simulink model "ASM_Traffic_V2X_Complete_Model_2"  (R2019a)
settings: Solver=ode1  StartTime=SIM.tstart.v  StopTime=Inf  FixedStep=SIM.StepSize.v  RelTol=1e-3
PostLoadFcn:
  | if any(exist('dsrtsu_mdlpostloadfcn', 'file') ~= 0), dsrtsu_mdlpostloadfcn('Execute', bdroot); end
  | try, asm_mdl_postloadfcn(bdroot, 'UpdateModel', 2200); catch, disp(lasterr); end,
undefined symbols (not defined in the file): _SensorPnts_1, _SensorPnts_13, _SensorPnts_17, _SensorPnts_21, _SensorPnts_25, _SensorPnts_29, _SensorPnts_33, _SensorPnts_37, _SensorPnts_41, _SensorPnts_45, _SensorPnts_49, _SensorPnts_5, _SensorPnts_53, _SensorPnts_57, _SensorPnts_9, _to_, CPT, G5A, ITS, MDL, rad, s_to_rpm, SIM
libraries: simulink x169, ASM_VehicleDynamics_lib x126, ASM_Traffic_lib x83, ASM_Utils_lib x49, mdbs x45, ASM_Environment_lib x17, dspindex x12, dsaV2xLibraryAux x10, dsmpblib x6, dsaV2xAsn1Library x4, dsaV2xLibrary x4, ASM_BrakeHydraulics_lib x4
(part 29 of 36)

== system ASM_Traffic_V2X_Complete_Model_2/MDL/Environment/Traffic/Sensors/Object_Sensor_3D/SensorMapping/NearestSurfaceMapping ==
  Sensor1_Signals[] : Inport
  Sensor2_Signals[] : Inport  Port=2
  Sensor3_Signals[] : Inport  Port=3
  NearestSurfaceSignals_Sensor1 : Subsystem
  NearestSurfaceSignals_Sensor2 : Subsystem
  NearestSurfaceSignals_Sensor3 : Subsystem
  Terminator{1..42} (42 alike) : Terminator
  wires:
  NearestSurfaceSignals_Sensor1/10(Pos_x_NearstSurfacePnt4_CoorSys_S[m]) -> Terminator42/1
  NearestSurfaceSignals_Sensor1/8(Pos_y_NearstSurfacePnt3_CoorSys_S[m]) -> Terminator12/1
  NearestSurfaceSignals_Sensor1/7(Pos_x_NearstSurfacePnt3_CoorSys_S[m]) -> Terminator11/1
  NearestSurfaceSignals_Sensor1/12(Pos_z_NearstSurfacePnt4_CoorSys_S[m]) -> Terminator4/1
  NearestSurfaceSignals_Sensor1/9(Pos_z_NearstSurfacePnt3_CoorSys_S[m]) -> Terminator13/1
  NearestSurfaceSignals_Sensor1/11(Pos_y_NearstSurfacePnt4_CoorSys_S[m]) -> Terminator3/1
  NearestSurfaceSignals_Sensor1/13(NearestSurf_Pnts_Index[]) -> Terminator5/1
  NearestSurfaceSignals_Sensor1/14(NearestSurf_Index[]) -> Terminator6/1
  NearestSurfaceSignals_Sensor1/1(Pos_x_NearstSurfacePnt1_CoorSys_S[m]) -> Terminator1/1
  NearestSurfaceSignals_Sensor1/6(Pos_z_NearstSurfacePnt2_CoorSys_S[m]) -> Terminator10/1
  NearestSurfaceSignals_Sensor1/5(Pos_y_NearstSurfacePnt2_CoorSys_S[m]) -> Terminator9/1
  NearestSurfaceSignals_Sensor1/2(Pos_y_NearstSurfacePnt1_CoorSys_S[m]) -> Terminator2/1
  NearestSurfaceSignals_Sensor1/4(Pos_x_NearstSurfacePnt2_CoorSys_S[m]) -> Terminator8/1
  NearestSurfaceSignals_Sensor1/3(Pos_z_NearstSurfacePnt1_CoorSys_S[m]) -> Terminator7/1
  NearestSurfaceSignals_Sensor3/10(Pos_x_NearstSurfacePnt4_CoorSys_S[m]) -> Terminator41/1
  NearestSurfaceSignals_Sensor3/8(Pos_y_NearstSurfacePnt3_CoorSys_S[m]) -> Terminator39/1
  NearestSurfaceSignals_Sensor3/7(Pos_x_NearstSurfacePnt3_CoorSys_S[m]) -> Terminator38/1
  NearestSurfaceSignals_Sensor3/12(Pos_z_NearstSurfacePnt4_CoorSys_S[m]) -> Terminator31/1
  NearestSurfaceSignals_Sensor3/9(Pos_z_NearstSurfacePnt3_CoorSys_S[m]) -> Terminator40/1
  NearestSurfaceSignals_Sensor3/11(Pos_y_NearstSurfacePnt4_CoorSys_S[m]) -> Terminator30/1
  NearestSurfaceSignals_Sensor3/13(NearestSurf_Pnts_Index[]) -> Terminator32/1
  NearestSurfaceSignals_Sensor3/14(NearestSurf_Index[]) -> Terminator33/1
  NearestSurfaceSignals_Sensor3/1(Pos_x_NearstSurfacePnt1_CoorSys_S[m]) -> Terminator28/1
  NearestSurfaceSignals_Sensor3/6(Pos_z_NearstSurfacePnt2_CoorSys_S[m]) -> Terminator37/1
  NearestSurfaceSignals_Sensor3/5(Pos_y_NearstSurfacePnt2_CoorSys_S[m]) -> Terminator36/1
  NearestSurfaceSignals_Sensor3/2(Pos_y_NearstSurfacePnt1_CoorSys_S[m]) -> Terminator29/1
  NearestSurfaceSignals_Sensor3/4(Pos_x_NearstSurfacePnt2_CoorSys_S[m]) -> Terminator35/1
  NearestSurfaceSignals_Sensor3/3(Pos_z_NearstSurfacePnt1_CoorSys_S[m]) -> Terminator34/1
  NearestSurfaceSignals_Sensor2/3(Pos_z_NearstSurfacePnt1_CoorSys_S[m]) -> Terminator20/1
  NearestSurfaceSignals_Sensor2/4(Pos_x_NearstSurfacePnt2_CoorSys_S[m]) -> Terminator21/1
  NearestSurfaceSignals_Sensor2/2(Pos_y_NearstSurfacePnt1_CoorSys_S[m]) -> Terminator15/1
  NearestSurfaceSignals_Sensor2/5(Pos_y_NearstSurfacePnt2_CoorSys_S[m]) -> Terminator22/1
  NearestSurfaceSignals_Sensor2/6(Pos_z_NearstSurfacePnt2_CoorSys_S[m]) -> Terminator23/1
  NearestSurfaceSignals_Sensor2/1(Pos_x_NearstSurfacePnt1_CoorSys_S[m]) -> Terminator14/1
  NearestSurfaceSignals_Sensor2/14(NearestSurf_Index[]) -> Terminator19/1
  NearestSurfaceSignals_Sensor2/13(NearestSurf_Pnts_Index[]) -> Terminator18/1
  Sensor2_Signals[]/1 -> NearestSurfaceSignals_Sensor2/1(SensorSignals[])
  Sensor3_Signals[]/1 -> NearestSurfaceSignals_Sensor3/1(SensorSignals[])
  Sensor1_Signals[]/1 -> NearestSurfaceSignals_Sensor1/1(SensorSignals[])
  NearestSurfaceSignals_Sensor2/11(Pos_y_NearstSurfacePnt4_CoorSys_S[m]) -> Terminator16/1
  NearestSurfaceSignals_Sensor2/9(Pos_z_NearstSurfacePnt3_CoorSys_S[m]) -> Terminator26/1
  NearestSurfaceSignals_Sensor2/12(Pos_z_NearstSurfacePnt4_CoorSys_S[m]) -> Terminator17/1
  NearestSurfaceSignals_Sensor2/7(Pos_x_NearstSurfacePnt3_CoorSys_S[m]) -> Terminator24/1
  NearestSurfaceSignals_Sensor2/8(Pos_y_NearstSurfacePnt3_CoorSys_S[m]) -> Terminator25/1
  NearestSurfaceSignals_Sensor2/10(Pos_x_NearstSurfacePnt4_CoorSys_S[m]) -> Terminator27/1

== system ASM_Traffic_V2X_Complete_Model_2/MDL/Environment/Traffic/Sensors/Object_Sensor_3D/SensorMapping/Signals_to_ACC_SoftECU ==
  Sensor_1_ACC_In : Inport
  Sensor_2_ACC_In : Inport  Port=2
  Bus Creator : BusCreator  Inputs=3
  Bus Creator1 : BusCreator  Inputs=2
  Bus Creator2 : BusCreator  Inputs=4
  Bus Selector : BusSelector  OutputSignals=SensorOutput.Dist_Object[m],SensorOutput.v_Rel_Object[m|s],SensorOutput.Angle_Hor_Object[deg]
  Bus Selector1 : BusSelector  OutputSignals=SensorOutput.Dist_Object[m],SensorOutput.v_Rel_Object[m|s],SensorOutput.Angle_Hor_Object[deg],SensorOutput.Object_ID[]
  Sensor_Signals : Outport
  wires:
  Bus Selector1/3 -> Bus Creator2/3  "<Angle_Hor_Object[deg]>"
  Bus Selector1/2 -> Bus Creator2/2  "<v_Rel_Object[m|s]>"
  Sensor_2_ACC_In/1 -> Bus Selector1/1
  Bus Selector1/4 -> Bus Creator2/4  "<Object_ID[]>"
  Bus Selector1/1 -> Bus Creator2/1  "<Dist_Object[m]>"
  Bus Creator2/1 -> Bus Creator1/2  "Sensor_2_ACC"
  Sensor_1_ACC_In/1 -> Bus Selector/1
  Bus Selector/1 -> Bus Creator/1  "<Dist_Object[m]>"
  Bus Selector/2 -> Bus Creator/2  "<v_Rel_Object[m|s]>"
  Bus Selector/3 -> Bus Creator/3  "<Angle_Hor_Object[deg]>"
  Bus Creator/1 -> Bus Creator1/1  "Sensor_1_ACC"
  Bus Creator1/1 -> Sensor_Signals/1  "SensorSignals"

== system ASM_Traffic_V2X_Complete_Model_2/MDL/Environment/Traffic/Sensors/Object_Sensor_3D/SensorParameters/ObjectSensor3DParameters_1 ==
  Demux : Demux  Outputs=3
  Demux1 : Demux  Outputs=3
  MODELDESK_GROUP : ASM_Utils_lib/ModelDeskInterface/MODELDESK_GROUP  MDLDGroup=Object Sensor 3D 1  ASMProperties=struct('Name','MODELDESK_GROUP','Version','1.0','Library','ASM_Utils_lib')
  Mux1 : Mux  Inputs=21
  OBJECT_SENSOR_3D_PARAMETERS_1 : ASM_Traffic_lib/Sensors/Object_Sensor_3D/OBJECT_SENSOR_3D_PARAMETERS  Tag=ASM_SUBCOMPONENT  Sw_Sensor_Enable=MDL.Traffic.Sensors.ObjectSensor3D_1.Sw_Sensor_Enable  Const_SensorIdx=MDL.Traffic.Sensors.ObjectSensor3D_1.Const_SensorIdx  Const_t_Offs_Sensor=MDL.Traffic.Sensors.ObjectSensor3D_1.Const_t_Offs_Sensor  Const_t_Cycle_Sensor=MDL.Traffic.Sensors.ObjectSensor3D_1.Const_t_Cycle_Sensor  Const_t_Delay_SensorOutput=MDL.Traffic.Sensors.ObjectSensor3D_1.Const_t_Delay_SensorOutput  Sw_Geometry=MDL.Traffic.Sensors.ObjectSensor3D_1.Sw_Geometry  Const_Pos_Sensor_Apex_CoorSys_V=MDL.Traffic.Sensors.ObjectSensor3D_1.Const_Pos_Sensor_Apex_CoorSys_V  Const_Angle_Orientation_Sensor_CoorSys_V=MDL.Traffic.Sensors.ObjectSensor3D_1.Const_Angle_Orientation_Sensor_CoorSys_V  Const_Length_ScopeZone=MDL.Traffic.Sensors.ObjectSensor3D_1.Const_Length_ScopeZone  Const_Angle_ScopeZone_Horizontal=MDL.Traffic.Sensors.ObjectSensor3D_1.Const_Angle_ScopeZone_Horizontal  Const_Angle_ScopeZone_Vertical=MDL.Traffic.Sensors.ObjectSensor3D_1.Const_Angle_ScopeZone_Vertical  Const_Length_ScopeZone_Head=MDL.Traffic.Sensors.ObjectSensor3D_1.Const_Length_ScopeZone_Head  Const_Length_BlindZone=MDL.Traffic.Sensors.ObjectSensor3D_1.Const_Length_BlindZone  Sw_Occlusion_Mode=MDL.Traffic.Sensors.ObjectSensor3D_1.Sw_Occlusion_Mode  Const_Threshold_Occlusion_Ratio=MDL.Traffic.Sensors.ObjectSensor3D_1.Const_Threshold_Occlusion_Ratio  Sw_Object_Points_Calculation_Enable=MDL.Traffic.Sensors.ObjectSensor3D_1.Sw_Object_Points_Calculation_Enable  Sw_Object_Points_Occlusion_Enable=MDL.Traffic.Sensors.ObjectSensor3D_1.Sw_Object_Points_Occlusion_Enable  ASMProperties=struct('Name','OBJECT_SENSOR_3D_PARAMETERS','Version','4.0','Library','ASM_Traffic_lib')  ASMInstanceName=object_sensor_3d_parameters  ASMInstanceID=1
  Sensor_Parameters[] : Outport
  tag scope: ASMBUS_Environment_Traffic_3DObjSensor1_Parameters=global
  wires:
  OBJECT_SENSOR_3D_PARAMETERS_1/18 -> Mux1/21
  OBJECT_SENSOR_3D_PARAMETERS_1/17 -> Mux1/20
  OBJECT_SENSOR_3D_PARAMETERS_1/16 -> Mux1/19
  OBJECT_SENSOR_3D_PARAMETERS_1/15 -> Mux1/18
  Demux1/3 -> Mux1/12
  Demux1/1 -> Mux1/10
  Demux1/2 -> Mux1/11
  Demux/3 -> Mux1/9
  Demux/2 -> Mux1/8
  Demux/1 -> Mux1/7
  OBJECT_SENSOR_3D_PARAMETERS_1/14 -> Mux1/17
  OBJECT_SENSOR_3D_PARAMETERS_1/11 -> Mux1/14
  OBJECT_SENSOR_3D_PARAMETERS_1/6 -> Mux1/5
  OBJECT_SENSOR_3D_PARAMETERS_1/5 -> Mux1/4
  OBJECT_SENSOR_3D_PARAMETERS_1/4 -> Mux1/3
  Mux1/1 -> Sensor_Parameters[]/1
  OBJECT_SENSOR_3D_PARAMETERS_1/10 -> Mux1/13
  OBJECT_SENSOR_3D_PARAMETERS_1/13 -> Mux1/16
  OBJECT_SENSOR_3D_PARAMETERS_1/9 -> Demux1/1
  OBJECT_SENSOR_3D_PARAMETERS_1/8 -> Demux/1
  OBJECT_SENSOR_3D_PARAMETERS_1/1 -> [ASMBUS_Environment_Traffic_3DObjSensor1_Parameters]
  OBJECT_SENSOR_3D_PARAMETERS_1/3 -> Mux1/2
  OBJECT_SENSOR_3D_PARAMETERS_1/2 -> Mux1/1
  OBJECT_SENSOR_3D_PARAMETERS_1/12 -> Mux1/15
  OBJECT_SENSOR_3D_PARAMETERS_1/7 -> Mux1/6

== system ASM_Traffic_V2X_Complete_Model_2/MDL/Environment/Traffic/Sensors/Object_Sensor_3D/SensorParameters/ObjectSensor3DParameters_2 ==
  Demux2 : Demux  Outputs=3
  Demux3 : Demux  Outputs=3
  MODELDESK_GROUP : ASM_Utils_lib/ModelDeskInterface/MODELDESK_GROUP  MDLDGroup=Object Sensor 3D 2  ASMProperties=struct('Name','MODELDESK_GROUP','Version','1.0','Library','ASM_Utils_lib')
  Mux : Mux  Inputs=21
  OBJECT_SENSOR_3D_PARAMETERS_2 : ASM_Traffic_lib/Sensors/Object_Sensor_3D/OBJECT_SENSOR_3D_PARAMETERS  Tag=ASM_SUBCOMPONENT  Sw_Sensor_Enable=MDL.Traffic.Sensors.ObjectSensor3D_2.Sw_Sensor_Enable  Const_SensorIdx=MDL.Traffic.Sensors.ObjectSensor3D_2.Const_SensorIdx  Const_t_Offs_Sensor=MDL.Traffic.Sensors.ObjectSensor3D_2.Const_t_Offs_Sensor  Const_t_Cycle_Sensor=MDL.Traffic.Sensors.ObjectSensor3D_2.Const_t_Cycle_Sensor  Const_t_Delay_SensorOutput=MDL.Traffic.Sensors.ObjectSensor3D_2.Const_t_Delay_SensorOutput  Sw_Geometry=MDL.Traffic.Sensors.ObjectSensor3D_2.Sw_Geometry  Const_Pos_Sensor_Apex_CoorSys_V=MDL.Traffic.Sensors.ObjectSensor3D_2.Const_Pos_Sensor_Apex_CoorSys_V  Const_Angle_Orientation_Sensor_CoorSys_V=MDL.Traffic.Sensors.ObjectSensor3D_2.Const_Angle_Orientation_Sensor_CoorSys_V  Const_Length_ScopeZone=MDL.Traffic.Sensors.ObjectSensor3D_2.Const_Length_ScopeZone  Const_Angle_ScopeZone_Horizontal=MDL.Traffic.Sensors.ObjectSensor3D_2.Const_Angle_ScopeZone_Horizontal  Const_Angle_ScopeZone_Vertical=MDL.Traffic.Sensors.ObjectSensor3D_2.Const_Angle_ScopeZone_Vertical  Const_Length_ScopeZone_Head=MDL.Traffic.Sensors.ObjectSensor3D_2.Const_Length_ScopeZone_Head  Const_Length_BlindZone=MDL.Traffic.Sensors.ObjectSensor3D_2.Const_Length_BlindZone  Sw_Occlusion_Mode=MDL.Traffic.Sensors.ObjectSensor3D_2.Sw_Occlusion_Mode  Const_Threshold_Occlusion_Ratio=MDL.Traffic.Sensors.ObjectSensor3D_2.Const_Threshold_Occlusion_Ratio  Sw_Object_Points_Calculation_Enable=MDL.Traffic.Sensors.ObjectSensor3D_2.Sw_Object_Points_Calculation_Enable  Sw_Object_Points_Occlusion_Enable=MDL.Traffic.Sensors.ObjectSensor3D_2.Sw_Object_Points_Occlusion_Enable  ASMProperties=struct('Name','OBJECT_SENSOR_3D_PARAMETERS','Version','4.0','Library','ASM_Traffic_lib')  ASMInstanceName=object_sensor_3d_parameters  ASMInstanceID=2
      settings: AttributesFormatString=Instance Name: object_sensor_3d_parameters\nInstance ID: 2
  Sensor_Parameters[] : Outport
  tag scope: ASMBUS_Environment_Traffic_3DObjSensor2_Parameters=global
  wires:
  OBJECT_SENSOR_3D_PARAMETERS_2/18 -> Mux/21
  OBJECT_SENSOR_3D_PARAMETERS_2/17 -> Mux/20
  OBJECT_SENSOR_3D_PARAMETERS_2/16 -> Mux/19
  OBJECT_SENSOR_3D_PARAMETERS_2/15 -> Mux/18
  Demux3/3 -> Mux/12
  Demux3/1 -> Mux/10
  Demux3/2 -> Mux/11
  Demux2/3 -> Mux/9
  Demux2/1 -> Mux/7
  Demux2/2 -> Mux/8
  Mux/1 -> Sensor_Parameters[]/1
  OBJECT_SENSOR_3D_PARAMETERS_2/14 -> Mux/17
  OBJECT_SENSOR_3D_PARAMETERS_2/12 -> Mux/15
  OBJECT_SENSOR_3D_PARAMETERS_2/1 -> [ASMBUS_Environment_Traffic_3DObjSensor2_Parameters]
  OBJECT_SENSOR_3D_PARAMETERS_2/9 -> Demux3/1
  OBJECT_SENSOR_3D_PARAMETERS_2/10 -> Mux/13
  OBJECT_SENSOR_3D_PARAMETERS_2/3 -> Mux/2
  OBJECT_SENSOR_3D_PARAMETERS_2/7 -> Mux/6
  OBJECT_SENSOR_3D_PARAMETERS_2/4 -> Mux/3
  OBJECT_SENSOR_3D_PARAMETERS_2/13 -> Mux/16
  OBJECT_SENSOR_3D_PARAMETERS_2/8 -> Demux2/1
  OBJECT_SENSOR_3D_PARAMETERS_2/6 -> Mux/5
  OBJECT_SENSOR_3D_PARAMETERS_2/11 -> Mux/14
  OBJECT_SENSOR_3D_PARAMETERS_2/2 -> Mux/1
  OBJECT_SENSOR_3D_PARAMETERS_2/5 -> Mux/4

== system ASM_Traffic_V2X_Complete_Model_2/MDL/Environment/Traffic/Sensors/Object_Sensor_3D/SensorParameters/ObjectSensor3DParameters_3 ==
  Demux4 : Demux  Outputs=3
  Demux5 : Demux  Outputs=3
  MODELDESK_GROUP : ASM_Utils_lib/ModelDeskInterface/MODELDESK_GROUP  MDLDGroup=Object Sensor 3D 3  ASMProperties=struct('Name','MODELDESK_GROUP','Version','1.0','Library','ASM_Utils_lib')
  Mux2 : Mux  Inputs=21
  OBJECT_SENSOR_3D_PARAMETERS_3 : ASM_Traffic_lib/Sensors/Object_Sensor_3D/OBJECT_SENSOR_3D_PARAMETERS  Tag=ASM_SUBCOMPONENT  Sw_Sensor_Enable=MDL.Traffic.Sensors.ObjectSensor3D_3.Sw_Sensor_Enable  Const_SensorIdx=MDL.Traffic.Sensors.ObjectSensor3D_3.Const_SensorIdx  Const_t_Offs_Sensor=MDL.Traffic.Sensors.ObjectSensor3D_3.Const_t_Offs_Sensor  Const_t_Cycle_Sensor=MDL.Traffic.Sensors.ObjectSensor3D_3.Const_t_Cycle_Sensor  Const_t_Delay_SensorOutput=MDL.Traffic.Sensors.ObjectSensor3D_3.Const_t_Delay_SensorOutput  Sw_Geometry=MDL.Traffic.Sensors.ObjectSensor3D_3.Sw_Geometry  Const_Pos_Sensor_Apex_CoorSys_V=MDL.Traffic.Sensors.ObjectSensor3D_3.Const_Pos_Sensor_Apex_CoorSys_V  Const_Angle_Orientation_Sensor_CoorSys_V=MDL.Traffic.Sensors.ObjectSensor3D_3.Const_Angle_Orientation_Sensor_CoorSys_V  Const_Length_ScopeZone=MDL.Traffic.Sensors.ObjectSensor3D_3.Const_Length_ScopeZone  Const_Angle_ScopeZone_Horizontal=MDL.Traffic.Sensors.ObjectSensor3D_3.Const_Angle_ScopeZone_Horizontal  Const_Angle_ScopeZone_Vertical=MDL.Traffic.Sensors.ObjectSensor3D_3.Const_Angle_ScopeZone_Vertical  Const_Length_ScopeZone_Head=MDL.Traffic.Sensors.ObjectSensor3D_3.Const_Length_ScopeZone_Head  Const_Length_BlindZone=MDL.Traffic.Sensors.ObjectSensor3D_3.Const_Length_BlindZone  Sw_Occlusion_Mode=MDL.Traffic.Sensors.ObjectSensor3D_3.Sw_Occlusion_Mode  Const_Threshold_Occlusion_Ratio=MDL.Traffic.Sensors.ObjectSensor3D_3.Const_Threshold_Occlusion_Ratio  Sw_Object_Points_Calculation_Enable=MDL.Traffic.Sensors.ObjectSensor3D_3.Sw_Object_Points_Calculation_Enable  Sw_Object_Points_Occlusion_Enable=MDL.Traffic.Sensors.ObjectSensor3D_3.Sw_Object_Points_Occlusion_Enable  ASMProperties=struct('Name','OBJECT_SENSOR_3D_PARAMETERS','Version','4.0','Library','ASM_Traffic_lib')  ASMInstanceName=object_sensor_3d_parameters  ASMInstanceID=3
      settings: AttributesFormatString=Instance Name: object_sensor_3d_parameters\nInstance ID: 3
  Sensor_Parameters[] : Outport
  tag scope: ASMBUS_Environment_Traffic_3DObjSensor3_Parameters=global
  wires:
  OBJECT_SENSOR_3D_PARAMETERS_3/18 -> Mux2/21
  OBJECT_SENSOR_3D_PARAMETERS_3/17 -> Mux2/20
  OBJECT_SENSOR_3D_PARAMETERS_3/16 -> Mux2/19
  OBJECT_SENSOR_3D_PARAMETERS_3/15 -> Mux2/18
  Demux5/3 -> Mux2/9
  Demux5/1 -> Mux2/7
  Demux5/2 -> Mux2/8
  Demux4/3 -> Mux2/12
  Demux4/1 -> Mux2/10
  Demux4/2 -> Mux2/11
  Mux2/1 -> Sensor_Parameters[]/1
  OBJECT_SENSOR_3D_PARAMETERS_3/14 -> Mux2/17
  OBJECT_SENSOR_3D_PARAMETERS_3/13 -> Mux2/16
  OBJECT_SENSOR_3D_PARAMETERS_3/12 -> Mux2/15
  OBJECT_SENSOR_3D_PARAMETERS_3/11 -> Mux2/14
  OBJECT_SENSOR_3D_PARAMETERS_3/10 -> Mux2/13
  OBJECT_SENSOR_3D_PARAMETERS_3/9 -> Demux4/1
  OBJECT_SENSOR_3D_PARAMETERS_3/8 -> Demux5/1
  OBJECT_SENSOR_3D_PARAMETERS_3/7 -> Mux2/6
  OBJECT_SENSOR_3D_PARAMETERS_3/6 -> Mux2/5
  OBJECT_SENSOR_3D_PARAMETERS_3/5 -> Mux2/4
  OBJECT_SENSOR_3D_PARAMETERS_3/4 -> Mux2/3
  OBJECT_SENSOR_3D_PARAMETERS_3/3 -> Mux2/2
  OBJECT_SENSOR_3D_PARAMETERS_3/2 -> Mux2/1
  OBJECT_SENSOR_3D_PARAMETERS_3/1 -> [ASMBUS_Environment_Traffic_3DObjSensor3_Parameters]

== system ASM_Traffic_V2X_Complete_Model_2/MDLUserInterface/Environment/MDL_DISP/Traffic/Fellow_Movement/GetFellowDataByIndex_1/SwitchFellowMovementData ==
  TrafficBus : Inport
  Switch : Inport  Port=2
  Bus Selector2 : BusSelector  OutputSignals=FellowMovement.TrafficScheduler.Flag_FellowsUsed[0|1]
  Bus Selector3 : BusSelector  OutputSignals=FellowMovement.FellowMovement.s_Fellows[m]
  Bus Selector4 : BusSelector  OutputSignals=FellowMovement.FellowMovement.d_Total_Fellows[m]
  Bus Selector5 : BusSelector  OutputSignals=FellowMovement.FellowMovement.v_Fellows[km|h]
  Flag_Fellow_Used[0|1] : Subsystem
      mask Display: disp('')
  Selector{,1..3} (4 alike) : Selector  InputPortWidth=MDL.Traffic.MaxNumFellows.v  IndexOptions=Index vector (port)  Indices=[1 3]  OutputSizes=1
  d_Total_Fellow[m] : Subsystem
      mask Display: disp('')
  s_Fellow[m] : Subsystem
      mask Display: disp('')
  v_Fellow[km|h] : Subsystem
      mask Display: disp('')
  "Flag_Fellow_Used[0|1] " : Outport
  "s_Fellow[m] " : Outport  Port=2
  "d_Total_Fellow[m] " : Outport  Port=3
  "v_Fellow[km|h] " : Outport  Port=4
  wires:
  Flag_Fellow_Used[0|1]/1(Out1) -> "Flag_Fellow_Used[0|1] "/1  "Flag_Fellow_Used[0|1]"
  s_Fellow[m]/1(Out1) -> "s_Fellow[m] "/1  "s_Fellow[m]"
  d_Total_Fellow[m]/1(Out1) -> "d_Total_Fellow[m] "/1  "d_Total_Fellow[m]"
  v_Fellow[km|h]/1(Out1) -> "v_Fellow[km|h] "/1  "v_Fellow[km|h]"
  Switch/1 -> Selector3/2, Selector2/2, Selector1/2, Selector/2
  Bus Selector2/1 -> Selector/1  "<Flag_FellowsUsed[0|1]>"
  Selector/1 -> Flag_Fellow_Used[0|1]/1(In1)
  Bus Selector3/1 -> Selector1/1  "<s_Fellows[m]>"
  Selector1/1 -> s_Fellow[m]/1(In1)
  Bus Selector4/1 -> Selector2/1  "<d_Total_Fellows[m]>"
  Selector2/1 -> d_Total_Fellow[m]/1(In1)
  Bus Selector5/1 -> Selector3/1  "<v_Fellows[km|h]>"
  Selector3/1 -> v_Fellow[km|h]/1(In1)
  TrafficBus/1 -> Bus Selector5/1, Bus Selector4/1, Bus Selector3/1, Bus Selector2/1

== system ASM_Traffic_V2X_Complete_Model_2/MDLUserInterface/Environment/MDL_DISP/Traffic/Fellow_Movement/GetFellowDataByIndex_1/SwitchInfoData ==
  TrafficBus : Inport
  Switch : Inport  Port=2
  Bus Selector1 : BusSelector  OutputSignals=FellowMovement.TrafficScheduler.Info.CurrentSegment_Fellows[]
  Bus Selector2 : BusSelector  OutputSignals=FellowMovement.TrafficScheduler.Info.t_local_Fellows[s]
  Bus Selector44 : BusSelector  OutputSignals=FellowMovement.TrafficScheduler.Info.CurrentSequence_Fellows[]
  Selector : Selector  InputPortWidth=MDL.Traffic.MaxNumFellows.v  IndexOptions=Index vector (port)  Indices=[1 3]  OutputSizes=1
  Selector1 : Selector  InputPortWidth=MDL.Traffic.MaxNumFellows.v  IndexOptions=Index vector (port)  Indices=[1 3]  OutputSizes=1
  Selector2 : Selector  InputPortWidth=MDL.Traffic.MaxNumFellows.v  IndexOptions=Index vector (port)  Indices=[1 3]  OutputSizes=1
  CurrentSequence[] : Outport
  CurrentSegment[] : Outport  Port=2
  t_local[s] : Outport  Port=3
  wires:
  Bus Selector2/1 -> Selector2/1  "<t_local_Fellows[s]>"
  TrafficBus/1 -> Bus Selector2/1, Bus Selector1/1, Bus Selector44/1
  Bus Selector1/1 -> Selector1/1  "<CurrentSegment_Fellows[]>"
  Selector1/1 -> CurrentSegment[]/1
  Bus Selector44/1 -> Selector/1  "<CurrentSequence_Fellows[]>"
  Selector/1 -> CurrentSequence[]/1
  Switch/1 -> Selector2/2, Selector1/2, Selector/2
  Selector2/1 -> t_local[s]/1

== system ASM_Traffic_V2X_Complete_Model_2/MDLUserInterface/Environment/MDL_DISP/Traffic/Fellow_Movement/GetFellowDataByIndex_2/SwitchFellowMovementData ==
  TrafficBus : Inport
  Switch : Inport  Port=2
  Bus Selector2 : BusSelector  OutputSignals=FellowMovement.TrafficScheduler.Flag_FellowsUsed[0|1]
  Bus Selector3 : BusSelector  OutputSignals=FellowMovement.FellowMovement.s_Fellows[m]
  Bus Selector4 : BusSelector  OutputSignals=FellowMovement.FellowMovement.d_Total_Fellows[m]
  Bus Selector5 : BusSelector  OutputSignals=FellowMovement.FellowMovement.v_Fellows[km|h]
  Flag_Fellow_Used[0|1] : Subsystem
      mask Display: disp('')
  Selector{,1..3} (4 alike) : Selector  InputPortWidth=MDL.Traffic.MaxNumFellows.v  IndexOptions=Index vector (port)  Indices=[1 3]  OutputSizes=1
  d_Total_Fellow[m] : Subsystem
      mask Display: disp('')
  s_Fellow[m] : Subsystem
      mask Display: disp('')
  v_Fellow[km|h] : Subsystem
      mask Display: disp('')
  "Flag_Fellow_Used[0|1] " : Outport
  "s_Fellow[m] " : Outport  Port=2
  "d_Total_Fellow[m] " : Outport  Port=3
  "v_Fellow[km|h] " : Outport  Port=4
  wires:
  TrafficBus/1 -> Bus Selector2/1, Bus Selector3/1, Bus Selector4/1, Bus Selector5/1
  Selector3/1 -> v_Fellow[km|h]/1(In1)
  Bus Selector5/1 -> Selector3/1  "<v_Fellows[km|h]>"
  Selector2/1 -> d_Total_Fellow[m]/1(In1)
  Bus Selector4/1 -> Selector2/1  "<d_Total_Fellows[m]>"
  Selector1/1 -> s_Fellow[m]/1(In1)
  Bus Selector3/1 -> Selector1/1  "<s_Fellows[m]>"
  Selector/1 -> Flag_Fellow_Used[0|1]/1(In1)
  Bus Selector2/1 -> Selector/1  "<Flag_FellowsUsed[0|1]>"
  Switch/1 -> Selector/2, Selector1/2, Selector2/2, Selector3/2
  v_Fellow[km|h]/1(Out1) -> "v_Fellow[km|h] "/1  "v_Fellow[km|h]"
  d_Total_Fellow[m]/1(Out1) -> "d_Total_Fellow[m] "/1  "d_Total_Fellow[m]"
  s_Fellow[m]/1(Out1) -> "s_Fellow[m] "/1  "s_Fellow[m]"
  Flag_Fellow_Used[0|1]/1(Out1) -> "Flag_Fellow_Used[0|1] "/1  "Flag_Fellow_Used[0|1]"

== system ASM_Traffic_V2X_Complete_Model_2/MDLUserInterface/Environment/MDL_DISP/Traffic/Fellow_Movement/GetFellowDataByIndex_2/SwitchInfoData ==
  TrafficBus : Inport
  Switch : Inport  Port=2
  Bus Selector1 : BusSelector  OutputSignals=FellowMovement.TrafficScheduler.Info.CurrentSegment_Fellows[]
  Bus Selector2 : BusSelector  OutputSignals=FellowMovement.TrafficScheduler.Info.t_local_Fellows[s]
  Bus Selector44 : BusSelector  OutputSignals=FellowMovement.TrafficScheduler.Info.CurrentSequence_Fellows[]
  Selector : Selector  InputPortWidth=MDL.Traffic.MaxNumFellows.v  IndexOptions=Index vector (port)  Indices=[1 3]  OutputSizes=1
  Selector1 : Selector  InputPortWidth=MDL.Traffic.MaxNumFellows.v  IndexOptions=Index vector (port)  Indices=[1 3]  OutputSizes=1
  Selector2 : Selector  InputPortWidth=MDL.Traffic.MaxNumFellows.v  IndexOptions=Index vector (port)  Indices=[1 3]  OutputSizes=1
  CurrentSequence[] : Outport
  CurrentSegment[] : Outport  Port=2
  t_local[s] : Outport  Port=3
  wires:
  Selector2/1 -> t_local[s]/1
  Switch/1 -> Selector/2, Selector1/2, Selector2/2
  Selector/1 -> CurrentSequence[]/1
  Bus Selector44/1 -> Selector/1  "<CurrentSequence_Fellows[]>"
  Selector1/1 -> CurrentSegment[]/1
  Bus Selector1/1 -> Selector1/1  "<CurrentSegment_Fellows[]>"
  TrafficBus/1 -> Bus Selector44/1, Bus Selector1/1, Bus Selector2/1
  Bus Selector2/1 -> Selector2/1  "<t_local_Fellows[s]>"

== system ASM_Traffic_V2X_Complete_Model_2/MDLUserInterface/Environment/MDL_DISP/Traffic/Fellow_Movement/GetFellowDataByIndex_3/SwitchFellowMovementData ==
  TrafficBus : Inport
  Switch : Inport  Port=2
  Bus Selector2 : BusSelector  OutputSignals=FellowMovement.TrafficScheduler.Flag_FellowsUsed[0|1]
  Bus Selector3 : BusSelector  OutputSignals=FellowMovement.FellowMovement.s_Fellows[m]
  Bus Selector4 : BusSelector  OutputSignals=FellowMovement.FellowMovement.d_Total_Fellows[m]
  Bus Selector5 : BusSelector  OutputSignals=FellowMovement.FellowMovement.v_Fellows[km|h]
  Flag_Fellow_Used[0|1] : Subsystem
      mask Display: disp('')
  Selector{,1..3} (4 alike) : Selector  InputPortWidth=MDL.Traffic.MaxNumFellows.v  IndexOptions=Index vector (port)  Indices=[1 3]  OutputSizes=1
  d_Total_Fellow[m] : Subsystem
      mask Display: disp('')
  s_Fellow[m] : Subsystem
      mask Display: disp('')
  v_Fellow[km|h] : Subsystem
      mask Display: disp('')
  "Flag_Fellow_Used[0|1] " : Outport
  "s_Fellow[m] " : Outport  Port=2
  "d_Total_Fellow[m] " : Outport  Port=3
  "v_Fellow[km|h] " : Outport  Port=4
  wires:
  Flag_Fellow_Used[0|1]/1(Out1) -> "Flag_Fellow_Used[0|1] "/1  "Flag_Fellow_Used[0|1]"
  s_Fellow[m]/1(Out1) -> "s_Fellow[m] "/1  "s_Fellow[m]"
  d_Total_Fellow[m]/1(Out1) -> "d_Total_Fellow[m] "/1  "d_Total_Fellow[m]"
  v_Fellow[km|h]/1(Out1) -> "v_Fellow[km|h] "/1  "v_Fellow[km|h]"
  Switch/1 -> Selector3/2, Selector2/2, Selector1/2, Selector/2
  Bus Selector2/1 -> Selector/1  "<Flag_FellowsUsed[0|1]>"
  Selector/1 -> Flag_Fellow_Used[0|1]/1(In1)
  Bus Selector3/1 -> Selector1/1  "<s_Fellows[m]>"
  Selector1/1 -> s_Fellow[m]/1(In1)
  Bus Selector4/1 -> Selector2/1  "<d_Total_Fellows[m]>"
  Selector2/1 -> d_Total_Fellow[m]/1(In1)
  Bus Selector5/1 -> Selector3/1  "<v_Fellows[km|h]>"
  Selector3/1 -> v_Fellow[km|h]/1(In1)
  TrafficBus/1 -> Bus Selector5/1, Bus Selector4/1, Bus Selector3/1, Bus Selector2/1

== system ASM_Traffic_V2X_Complete_Model_2/MDLUserInterface/Environment/MDL_DISP/Traffic/Fellow_Movement/GetFellowDataByIndex_3/SwitchInfoData ==
  TrafficBus : Inport
  Switch : Inport  Port=2
  Bus Selector1 : BusSelector  OutputSignals=FellowMovement.TrafficScheduler.Info.CurrentSegment_Fellows[]
  Bus Selector2 : BusSelector  OutputSignals=FellowMovement.TrafficScheduler.Info.t_local_Fellows[s]
  Bus Selector44 : BusSelector  OutputSignals=FellowMovement.TrafficScheduler.Info.CurrentSequence_Fellows[]
  Selector : Selector  InputPortWidth=MDL.Traffic.MaxNumFellows.v  IndexOptions=Index vector (port)  Indices=[1 3]  OutputSizes=1
  Selector1 : Selector  InputPortWidth=MDL.Traffic.MaxNumFellows.v  IndexOptions=Index vector (port)  Indices=[1 3]  OutputSizes=1
  Selector2 : Selector  InputPortWidth=MDL.Traffic.MaxNumFellows.v  IndexOptions=Index vector (port)  Indices=[1 3]  OutputSizes=1
  CurrentSequence[] : Outport
  CurrentSegment[] : Outport  Port=2
  t_local[s] : Outport  Port=3
  wires:
  Bus Selector2/1 -> Selector2/1  "<t_local_Fellows[s]>"
  TrafficBus/1 -> Bus Selector2/1, Bus Selector1/1, Bus Selector44/1
  Bus Selector1/1 -> Selector1/1  "<CurrentSegment_Fellows[]>"
  Selector1/1 -> CurrentSegment[]/1
  Bus Selector44/1 -> Selector/1  "<CurrentSequence_Fellows[]>"
  Selector/1 -> CurrentSequence[]/1
  Switch/1 -> Selector2/2, Selector1/2, Selector/2
  Selector2/1 -> t_local[s]/1

== system ASM_Traffic_V2X_Complete_Model_2/MDLUserInterface/Environment/MDL_DISP/Traffic/Object_Sensor_2D/IdxSelect_2DSensor/Scopezone_Element_Data_Selection1 ==
  Scopezone_El_Idx[1_60] : Inport
  Flag_Object_In_Scope[0Out|1In] : Inport  Port=2
  Flag_Sensor_Apex_In_Object[0Out|1In] : Inport  Port=3
  Angle_Hor_Rel[deg] : Inport  Port=4
  Object_ID[] : Inport  Port=5
  Object_Type[] : Inport  Port=6
  Distance[m] : Inport  Port=7
  v_Rel[m|s] : Inport  Port=8
  a_Rel[m|s2] : Inport  Port=9
  Height_Min[m] : Inport  Port=10
  Height_Max[m] : Inport  Port=11
  Angle_Hor_Rel[deg]1 : Subsystem
      mask Display: disp('')
  Distance[m]1 : Subsystem
      mask Display: disp('')
  Flag_Object_In_Scope[0Out|1In]1 : Subsystem
      mask Display: disp('')
  Flag_Sensor_Apex_In_Object[0Out|1In]1 : Subsystem
      mask Display: disp('')
  Height_Max[m]1 : Subsystem
      mask Display: disp('')
  Height_Min[m]1 : Subsystem
      mask Display: disp('')
  Object_ID[]1 : Subsystem
      mask Display: disp('')
  Object_Type[]1 : Subsystem
      mask Display: disp('')
  Selector{3..10} (8 alike) : Selector  InputPortWidth=MDL.Traffic.Sensors.ObjectSensor2D_Calculation.Const_Sensor_Output_Dimension.v  IndexOptions=Index vector (port)  Indices=[1 3]  OutputSizes=1
  Terminator_{1..10} (10 alike) : Terminator
  a_Rel[m|s2]1 : Subsystem
      mask Display: disp('')
  v_Rel[m|s]1 : Subsystem
      mask Display: disp('')
  wires:
  Selector5/1 -> Object_Type[]1/1(In1)
  Object_Type[]1/1(Out1) -> Terminator_5/1
  Selector4/1 -> Object_ID[]1/1(In1)
  Selector6/1 -> Distance[m]1/1(In1)
  Selector3/1 -> Angle_Hor_Rel[deg]1/1(In1)
  Selector7/1 -> v_Rel[m|s]1/1(In1)
  Selector8/1 -> a_Rel[m|s2]1/1(In1)
  Flag_Sensor_Apex_In_Object[0Out|1In]/1 -> Flag_Sensor_Apex_In_Object[0Out|1In]1/1(In1)
  Selector9/1 -> Height_Min[m]1/1(In1)
  Selector10/1 -> Height_Max[m]1/1(In1)
  Scopezone_El_Idx[1_60]/1 -> Selector3/2, Selector4/2, Selector5/2, Selector6/2, Selector7/2, Selector8/2, Selector9/2, Selector10/2
  Flag_Object_In_Scope[0Out|1In]/1 -> Flag_Object_In_Scope[0Out|1In]1/1(In1)
  Height_Max[m]1/1(Out1) -> Terminator_10/1
  Flag_Object_In_Scope[0Out|1In]1/1(Out1) -> Terminator_4/1
  Object_ID[]/1 -> Selector4/1
  Flag_Sensor_Apex_In_Object[0Out|1In]1/1(Out1) -> Terminator_1/1
  Angle_Hor_Rel[deg]1/1(Out1) -> Terminator_2/1
  a_Rel[m|s2]/1 -> Selector8/1
  Object_ID[]1/1(Out1) -> Terminator_3/1
  Object_Type[]/1 -> Selector5/1
  Height_Max[m]/1 -> Selector10/1
  Distance[m]/1 -> Selector6/1
  Angle_Hor_Rel[deg]/1 -> Selector3/1
  Height_Min[m]/1 -> Selector9/1
  Height_Min[m]1/1(Out1) -> Terminator_9/1
  a_Rel[m|s2]1/1(Out1) -> Terminator_8/1
  v_Rel[m|s]1/1(Out1) -> Terminator_7/1
  v_Rel[m|s]/1 -> Selector7/1
  Distance[m]1/1(Out1) -> Terminator_6/1

== system ASM_Traffic_V2X_Complete_Model_2/MDLUserInterface/Environment/MDL_DISP/Traffic/Object_Sensor_2D/IdxSelect_2DSensor/Scopezone_Element_Data_Selection2 ==
  Scopezone_El_Idx[1_60] : Inport
  Flag_Object_In_Scope[0Out|1In] : Inport  Port=2
  Flag_Sensor_Apex_In_Object[0Out|1In] : Inport  Port=3
  Angle_Hor_Rel[deg] : Inport  Port=4
  Object_ID[] : Inport  Port=5
  Object_Type[] : Inport  Port=6
  Distance[m] : Inport  Port=7
  v_Rel[m|s] : Inport  Port=8
  a_Rel[m|s2] : Inport  Port=9
  Height_Min[m] : Inport  Port=10
  Height_Max[m] : Inport  Port=11
  Angle_Hor_Rel[deg]1 : Subsystem
      mask Display: disp('')
  Distance[m]1 : Subsystem
      mask Display: disp('')
  Flag_Object_In_Scope[0Out|1In]1 : Subsystem
      mask Display: disp('')
  Flag_Sensor_Apex_In_Object[0Out|1In]1 : Subsystem
      mask Display: disp('')
  Height_Max[m]1 : Subsystem
      mask Display: disp('')
  Height_Min[m]1 : Subsystem
      mask Display: disp('')
  Object_ID[]1 : Subsystem
      mask Display: disp('')
  Object_Type[]1 : Subsystem
      mask Display: disp('')
  Selector{3..10} (8 alike) : Selector  InputPortWidth=MDL.Traffic.Sensors.ObjectSensor2D_Calculation.Const_Sensor_Output_Dimension.v  IndexOptions=Index vector (port)  Indices=[1 3]  OutputSizes=1
  Terminator_{1..10} (10 alike) : Terminator
  a_Rel[m|s2]1 : Subsystem
      mask Display: disp('')
  v_Rel[m|s]1 : Subsystem
      mask Display: disp('')
  wires:
  Distance[m]1/1(Out1) -> Terminator_6/1
  v_Rel[m|s]/1 -> Selector7/1
  v_Rel[m|s]1/1(Out1) -> Terminator_7/1
  a_Rel[m|s2]1/1(Out1) -> Terminator_8/1
  Height_Min[m]1/1(Out1) -> Terminator_9/1
  Height_Min[m]/1 -> Selector9/1
  Angle_Hor_Rel[deg]/1 -> Selector3/1
  Distance[m]/1 -> Selector6/1
  Height_Max[m]/1 -> Selector10/1
  Object_Type[]/1 -> Selector5/1
  Object_ID[]1/1(Out1) -> Terminator_3/1
  a_Rel[m|s2]/1 -> Selector8/1
  Angle_Hor_Rel[deg]1/1(Out1) -> Terminator_2/1
  Flag_Sensor_Apex_In_Object[0Out|1In]1/1(Out1) -> Terminator_1/1
  Object_ID[]/1 -> Selector4/1
  Flag_Object_In_Scope[0Out|1In]1/1(Out1) -> Terminator_4/1
  Height_Max[m]1/1(Out1) -> Terminator_10/1
  Flag_Object_In_Scope[0Out|1In]/1 -> Flag_Object_In_Scope[0Out|1In]1/1(In1)
  Scopezone_El_Idx[1_60]/1 -> Selector10/2, Selector9/2, Selector8/2, Selector7/2, Selector6/2, Selector5/2, Selector4/2, Selector3/2
  Selector10/1 -> Height_Max[m]1/1(In1)
  Selector9/1 -> Height_Min[m]1/1(In1)
  Flag_Sensor_Apex_In_Object[0Out|1In]/1 -> Flag_Sensor_Apex_In_Object[0Out|1In]1/1(In1)
  Selector8/1 -> a_Rel[m|s2]1/1(In1)
  Selector7/1 -> v_Rel[m|s]1/1(In1)
  Selector3/1 -> Angle_Hor_Rel[deg]1/1(In1)
  Selector6/1 -> Distance[m]1/1(In1)
  Selector4/1 -> Object_ID[]1/1(In1)
  Object_Type[]1/1(Out1) -> Terminator_5/1
  Selector5/1 -> Object_Type[]1/1(In1)

== system ASM_Traffic_V2X_Complete_Model_2/MDLUserInterface/Environment/MDL_DISP/Traffic/Object_Sensor_2D/IdxSelect_2DSensor/Scopezone_Element_Data_Selection3 ==
  Scopezone_El_Idx[1_60] : Inport
  Flag_Object_In_Scope[0Out|1In] : Inport  Port=2
  Flag_Sensor_Apex_In_Object[0Out|1In] : Inport  Port=3
  Angle_Hor_Rel[deg] : Inport  Port=4
  Object_ID[] : Inport  Port=5
  Object_Type[] : Inport  Port=6
  Distance[m] : Inport  Port=7
  v_Rel[m|s] : Inport  Port=8
  a_Rel[m|s2] : Inport  Port=9
  Height_Min[m] : Inport  Port=10
  Height_Max[m] : Inport  Port=11
  Angle_Hor_Rel[deg]1 : Subsystem
      mask Display: disp('')
  Distance[m]1 : Subsystem
      mask Display: disp('')
  Flag_Object_In_Scope[0Out|1In]1 : Subsystem
      mask Display: disp('')
  Flag_Sensor_Apex_In_Object[0Out|1In]1 : Subsystem
      mask Display: disp('')
  Height_Max[m]1 : Subsystem
      mask Display: disp('')
  Height_Min[m]1 : Subsystem
      mask Display: disp('')
  Object_ID[]1 : Subsystem
      mask Display: disp('')
  Object_Type[]1 : Subsystem
      mask Display: disp('')
  Selector{3..10} (8 alike) : Selector  InputPortWidth=MDL.Traffic.Sensors.ObjectSensor2D_Calculation.Const_Sensor_Output_Dimension.v  IndexOptions=Index vector (port)  Indices=[1 3]  OutputSizes=1
  Terminator_{1..10} (10 alike) : Terminator
  a_Rel[m|s2]1 : Subsystem
      mask Display: disp('')
  v_Rel[m|s]1 : Subsystem
      mask Display: disp('')
  wires:
  Selector5/1 -> Object_Type[]1/1(In1)
  Object_Type[]1/1(Out1) -> Terminator_5/1
  Selector4/1 -> Object_ID[]1/1(In1)
  Selector6/1 -> Distance[m]1/1(In1)
  Selector3/1 -> Angle_Hor_Rel[deg]1/1(In1)
  Selector7/1 -> v_Rel[m|s]1/1(In1)
  Selector8/1 -> a_Rel[m|s2]1/1(In1)
  Flag_Sensor_Apex_In_Object[0Out|1In]/1 -> Flag_Sensor_Apex_In_Object[0Out|1In]1/1(In1)
  Selector9/1 -> Height_Min[m]1/1(In1)
  Selector10/1 -> Height_Max[m]1/1(In1)
  Scopezone_El_Idx[1_60]/1 -> Selector3/2, Selector4/2, Selector5/2, Selector6/2, Selector7/2, Selector8/2, Selector9/2, Selector10/2
  Flag_Object_In_Scope[0Out|1In]/1 -> Flag_Object_In_Scope[0Out|1In]1/1(In1)
  Height_Max[m]1/1(Out1) -> Terminator_10/1
  Flag_Object_In_Scope[0Out|1In]1/1(Out1) -> Terminator_4/1
  Object_ID[]/1 -> Selector4/1
  Flag_Sensor_Apex_In_Object[0Out|1In]1/1(Out1) -> Terminator_1/1
  Angle_Hor_Rel[deg]1/1(Out1) -> Terminator_2/1
  a_Rel[m|s2]/1 -> Selector8/1
  Object_ID[]1/1(Out1) -> Terminator_3/1
  Object_Type[]/1 -> Selector5/1
  Height_Max[m]/1 -> Selector10/1
  Distance[m]/1 -> Selector6/1
  Angle_Hor_Rel[deg]/1 -> Selector3/1
  Height_Min[m]/1 -> Selector9/1
  Height_Min[m]1/1(Out1) -> Terminator_9/1
  a_Rel[m|s2]1/1(Out1) -> Terminator_8/1
  v_Rel[m|s]1/1(Out1) -> Terminator_7/1
  v_Rel[m|s]/1 -> Selector7/1
  Distance[m]1/1(Out1) -> Terminator_6/1

== system ASM_Traffic_V2X_Complete_Model_2/MDLUserInterface/Environment/MDL_DISP/Traffic/Object_Sensor_2D/IdxSelect_2DSensor/Scopezone_Element_Data_Selection4 ==
  Scopezone_El_Idx[1_60] : Inport
  Flag_Object_In_Scope[0Out|1In] : Inport  Port=2
  Flag_Sensor_Apex_In_Object[0Out|1In] : Inport  Port=3
  Angle_Hor_Rel[deg] : Inport  Port=4
  Object_ID[] : Inport  Port=5
  Object_Type[] : Inport  Port=6
  Distance[m] : Inport  Port=7
  v_Rel[m|s] : Inport  Port=8
  a_Rel[m|s2] : Inport  Port=9
  Height_Min[m] : Inport  Port=10
  Height_Max[m] : Inport  Port=11
  Angle_Hor_Rel[deg]1 : Subsystem
      mask Display: disp('')
  Distance[m]1 : Subsystem
      mask Display: disp('')
  Flag_Object_In_Scope[0Out|1In]1 : Subsystem
      mask Display: disp('')
  Flag_Sensor_Apex_In_Object[0Out|1In]1 : Subsystem
      mask Display: disp('')
  Height_Max[m]1 : Subsystem
      mask Display: disp('')
  Height_Min[m]1 : Subsystem
      mask Display: disp('')
  Object_ID[]1 : Subsystem
      mask Display: disp('')
  Object_Type[]1 : Subsystem
      mask Display: disp('')
  Selector{3..10} (8 alike) : Selector  InputPortWidth=MDL.Traffic.Sensors.ObjectSensor2D_Calculation.Const_Sensor_Output_Dimension.v  IndexOptions=Index vector (port)  Indices=[1 3]  OutputSizes=1
  Terminator_{1..10} (10 alike) : Terminator
  a_Rel[m|s2]1 : Subsystem
      mask Display: disp('')
  v_Rel[m|s]1 : Subsystem
      mask Display: disp('')
  wires:
  Distance[m]1/1(Out1) -> Terminator_6/1
  v_Rel[m|s]/1 -> Selector7/1
  v_Rel[m|s]1/1(Out1) -> Terminator_7/1
  a_Rel[m|s2]1/1(Out1) -> Terminator_8/1
  Height_Min[m]1/1(Out1) -> Terminator_9/1
  Height_Min[m]/1 -> Selector9/1
  Angle_Hor_Rel[deg]/1 -> Selector3/1
  Distance[m]/1 -> Selector6/1
  Height_Max[m]/1 -> Selector10/1
  Object_Type[]/1 -> Selector5/1
  Object_ID[]1/1(Out1) -> Terminator_3/1
  a_Rel[m|s2]/1 -> Selector8/1
  Angle_Hor_Rel[deg]1/1(Out1) -> Terminator_2/1
  Flag_Sensor_Apex_In_Object[0Out|1In]1/1(Out1) -> Terminator_1/1
  Object_ID[]/1 -> Selector4/1
  Flag_Object_In_Scope[0Out|1In]1/1(Out1) -> Terminator_4/1
  Height_Max[m]1/1(Out1) -> Terminator_10/1
  Flag_Object_In_Scope[0Out|1In]/1 -> Flag_Object_In_Scope[0Out|1In]1/1(In1)
  Scopezone_El_Idx[1_60]/1 -> Selector10/2, Selector9/2, Selector8/2, Selector7/2, Selector6/2, Selector5/2, Selector4/2, Selector3/2
  Selector10/1 -> Height_Max[m]1/1(In1)
  Selector9/1 -> Height_Min[m]1/1(In1)
  Flag_Sensor_Apex_In_Object[0Out|1In]/1 -> Flag_Sensor_Apex_In_Object[0Out|1In]1/1(In1)
  Selector8/1 -> a_Rel[m|s2]1/1(In1)
  Selector7/1 -> v_Rel[m|s]1/1(In1)
  Selector3/1 -> Angle_Hor_Rel[deg]1/1(In1)
  Selector6/1 -> Distance[m]1/1(In1)
  Selector4/1 -> Object_ID[]1/1(In1)
  Object_Type[]1/1(Out1) -> Terminator_5/1
  Selector5/1 -> Object_Type[]1/1(In1)

== system ASM_Traffic_V2X_Complete_Model_2/MDLUserInterface/Environment/MDL_DISP/Traffic/Object_Sensor_2D/IdxSelect_2DSensor/Scopezone_Element_Data_Selection5 ==
  Scopezone_El_Idx[1_60] : Inport
  Flag_Object_In_Scope[0Out|1In] : Inport  Port=2
  Flag_Sensor_Apex_In_Object[0Out|1In] : Inport  Port=3
  Angle_Hor_Rel[deg] : Inport  Port=4
  Object_ID[] : Inport  Port=5
  Object_Type[] : Inport  Port=6
  Distance[m] : Inport  Port=7
  v_Rel[m|s] : Inport  Port=8
  a_Rel[m|s2] : Inport  Port=9
  Height_Min[m] : Inport  Port=10
  Height_Max[m] : Inport  Port=11
  Angle_Hor_Rel[deg]1 : Subsystem
      mask Display: disp('')
  Distance[m]1 : Subsystem
      mask Display: disp('')
  Flag_Object_In_Scope[0Out|1In]1 : Subsystem
      mask Display: disp('')
  Flag_Sensor_Apex_In_Object[0Out|1In]1 : Subsystem
      mask Display: disp('')
  Height_Max[m]1 : Subsystem
      mask Display: disp('')
  Height_Min[m]1 : Subsystem
      mask Display: disp('')
  Object_ID[]1 : Subsystem
      mask Display: disp('')
  Object_Type[]1 : Subsystem
      mask Display: disp('')
  Selector{3..10} (8 alike) : Selector  InputPortWidth=MDL.Traffic.Sensors.ObjectSensor2D_Calculation.Const_Sensor_Output_Dimension.v  IndexOptions=Index vector (port)  Indices=[1 3]  OutputSizes=1
  Terminator_{1..10} (10 alike) : Terminator
  a_Rel[m|s2]1 : Subsystem
      mask Display: disp('')
  v_Rel[m|s]1 : Subsystem
      mask Display: disp('')
  wires:
  Selector5/1 -> Object_Type[]1/1(In1)
  Object_Type[]1/1(Out1) -> Terminator_5/1
  Selector4/1 -> Object_ID[]1/1(In1)
  Selector6/1 -> Distance[m]1/1(In1)
  Selector3/1 -> Angle_Hor_Rel[deg]1/1(In1)
  Selector7/1 -> v_Rel[m|s]1/1(In1)
  Selector8/1 -> a_Rel[m|s2]1/1(In1)
  Flag_Sensor_Apex_In_Object[0Out|1In]/1 -> Flag_Sensor_Apex_In_Object[0Out|1In]1/1(In1)
  Selector9/1 -> Height_Min[m]1/1(In1)
  Selector10/1 -> Height_Max[m]1/1(In1)
  Scopezone_El_Idx[1_60]/1 -> Selector3/2, Selector4/2, Selector5/2, Selector6/2, Selector7/2, Selector8/2, Selector9/2, Selector10/2
  Flag_Object_In_Scope[0Out|1In]/1 -> Flag_Object_In_Scope[0Out|1In]1/1(In1)
  Height_Max[m]1/1(Out1) -> Terminator_10/1
  Flag_Object_In_Scope[0Out|1In]1/1(Out1) -> Terminator_4/1
  Object_ID[]/1 -> Selector4/1
  Flag_Sensor_Apex_In_Object[0Out|1In]1/1(Out1) -> Terminator_1/1
  Angle_Hor_Rel[deg]1/1(Out1) -> Terminator_2/1
  a_Rel[m|s2]/1 -> Selector8/1
  Object_ID[]1/1(Out1) -> Terminator_3/1
  Object_Type[]/1 -> Selector5/1
  Height_Max[m]/1 -> Selector10/1
  Distance[m]/1 -> Selector6/1
  Angle_Hor_Rel[deg]/1 -> Selector3/1
  Height_Min[m]/1 -> Selector9/1
  Height_Min[m]1/1(Out1) -> Terminator_9/1
  a_Rel[m|s2]1/1(Out1) -> Terminator_8/1
  v_Rel[m|s]1/1(Out1) -> Terminator_7/1
  v_Rel[m|s]/1 -> Selector7/1
  Distance[m]1/1(Out1) -> Terminator_6/1

== system ASM_Traffic_V2X_Complete_Model_2/MDLUserInterface/Environment/MDL_DISP/Traffic/Object_Sensor_2D/Object_Sensor_2D_VisualizationData/Sensor_1_Front_Long ==
  Sensor : Inport
  Angle_Hor_Rel[deg] : Gain
  Angle_ScopeZone_Horizontal[deg] : Gain
  Angle_z_Orientation_Sensor_CoorSys_V[deg] : Gain
  Bus Selector : BusSelector  OutputSignals=Parameters.Sensor_Enable[0Off|1On],Parameters.Sensor_Detection_Mode[1Ray|2Sector],Parameters.Length_ScopeZone[m],Parameters.Pos_Sensor_Apex_CoorSys_V[x;y;z][m],Parameters.Angle_z_Orientation_Sensor_CoorSys_V[deg],Parameters.Angle_ScopeZone_Horizontal[deg],Parameters.SensorIdx[],SensorOutput.Object_ID[],SensorOutput.Distance[m],SensorOutput.Angle_Hor_Rel[deg]
  Distance[m] : Gain
  Length_ScopeZone[m] : Gain
  Object_ID[] : Gain
  Pos_Sensor_Apex_CoorSys_V[x;y;z][m] : Gain
  SensorIdx[] : Gain
  Sensor_Detection_Mode[1Ray|2Sector] : Gain
  Sensor_Enable[0Off|1On] : Gain
  Terminator{,1..9} (10 alike) : Terminator
  wires:
  Bus Selector/3 -> Length_ScopeZone[m]/1  "<Length_ScopeZone[m]>"
  Length_ScopeZone[m]/1 -> Terminator9/1
  Bus Selector/10 -> Angle_Hor_Rel[deg]/1  "<Angle_Hor_Rel[deg]>"
  Bus Selector/9 -> Distance[m]/1  "<Distance[m]>"
  Bus Selector/8 -> Object_ID[]/1  "<Object_ID[]>"
  Bus Selector/7 -> SensorIdx[]/1  "<SensorIdx[]>"
  Bus Selector/6 -> Angle_ScopeZone_Horizontal[deg]/1  "<Angle_ScopeZone_Horizontal[deg]>"
  Bus Selector/5 -> Angle_z_Orientation_Sensor_CoorSys_V[deg]/1  "<Angle_z_Orientation_Sensor_CoorSys_V[deg]>"
  Bus Selector/4 -> Pos_Sensor_Apex_CoorSys_V[x;y;z][m]/1  "<Pos_Sensor_Apex_CoorSys_V[x;y;z][m]>"
  Angle_Hor_Rel[deg]/1 -> Terminator8/1
  Distance[m]/1 -> Terminator7/1
  Object_ID[]/1 -> Terminator6/1
  SensorIdx[]/1 -> Terminator5/1
  Angle_ScopeZone_Horizontal[deg]/1 -> Terminator4/1
  Angle_z_Orientation_Sensor_CoorSys_V[deg]/1 -> Terminator3/1
  Pos_Sensor_Apex_CoorSys_V[x;y;z][m]/1 -> Terminator2/1
  Bus Selector/2 -> Sensor_Detection_Mode[1Ray|2Sector]/1  "<Sensor_Detection_Mode[1Ray|2Sector]>"
  Sensor_Detection_Mode[1Ray|2Sector]/1 -> Terminator1/1
  Sensor_Enable[0Off|1On]/1 -> Terminator/1
  Bus Selector/1 -> Sensor_Enable[0Off|1On]/1  "<Sensor_Enable[0Off|1On]>"
  Sensor/1 -> Bus Selector/1

== system ASM_Traffic_V2X_Complete_Model_2/MDLUserInterface/Environment/MDL_DISP/Traffic/Object_Sensor_2D/Object_Sensor_2D_VisualizationData/Sensor_2_Front_Left ==
  Sensor : Inport
  Angle_Hor_Rel[deg] : Gain
  Angle_ScopeZone_Horizontal[deg] : Gain
  Angle_z_Orientation_Sensor_CoorSys_V[deg] : Gain
  Bus Selector : BusSelector  OutputSignals=Parameters.Sensor_Enable[0Off|1On],Parameters.Sensor_Detection_Mode[1Ray|2Sector],Parameters.Length_ScopeZone[m],Parameters.Pos_Sensor_Apex_CoorSys_V[x;y;z][m],Parameters.Angle_z_Orientation_Sensor_CoorSys_V[deg],Parameters.Angle_ScopeZone_Horizontal[deg],Parameters.SensorIdx[],SensorOutput.Object_ID[],SensorOutput.Distance[m],SensorOutput.Angle_Hor_Rel[deg]
  Distance[m] : Gain
  Length_ScopeZone[m] : Gain
  Object_ID[] : Gain
  Pos_Sensor_Apex_CoorSys_V[x;y;z][m] : Gain
  SensorIdx[] : Gain
  Sensor_Detection_Mode[1Ray|2Sector] : Gain
  Sensor_Enable[0Off|1On] : Gain
  Terminator{,1..9} (10 alike) : Terminator
  wires:
  Sensor/1 -> Bus Selector/1
  Bus Selector/1 -> Sensor_Enable[0Off|1On]/1  "<Sensor_Enable[0Off|1On]>"
  Sensor_Enable[0Off|1On]/1 -> Terminator/1
  Sensor_Detection_Mode[1Ray|2Sector]/1 -> Terminator1/1
  Bus Selector/2 -> Sensor_Detection_Mode[1Ray|2Sector]/1  "<Sensor_Detection_Mode[1Ray|2Sector]>"
  Pos_Sensor_Apex_CoorSys_V[x;y;z][m]/1 -> Terminator2/1
  Angle_z_Orientation_Sensor_CoorSys_V[deg]/1 -> Terminator3/1
  Angle_ScopeZone_Horizontal[deg]/1 -> Terminator4/1
  SensorIdx[]/1 -> Terminator5/1
  Object_ID[]/1 -> Terminator6/1
  Distance[m]/1 -> Terminator7/1
  Angle_Hor_Rel[deg]/1 -> Terminator8/1
  Bus Selector/4 -> Pos_Sensor_Apex_CoorSys_V[x;y;z][m]/1  "<Pos_Sensor_Apex_CoorSys_V[x;y;z][m]>"
  Bus Selector/5 -> Angle_z_Orientation_Sensor_CoorSys_V[deg]/1  "<Angle_z_Orientation_Sensor_CoorSys_V[deg]>"
  Bus Selector/6 -> Angle_ScopeZone_Horizontal[deg]/1  "<Angle_ScopeZone_Horizontal[deg]>"
  Bus Selector/7 -> SensorIdx[]/1  "<SensorIdx[]>"
  Bus Selector/8 -> Object_ID[]/1  "<Object_ID[]>"
  Bus Selector/9 -> Distance[m]/1  "<Distance[m]>"
  Bus Selector/10 -> Angle_Hor_Rel[deg]/1  "<Angle_Hor_Rel[deg]>"
  Length_ScopeZone[m]/1 -> Terminator9/1
  Bus Selector/3 -> Length_ScopeZone[m]/1  "<Length_ScopeZone[m]>"

== system ASM_Traffic_V2X_Complete_Model_2/MDLUserInterface/Environment/MDL_DISP/Traffic/Object_Sensor_2D/Object_Sensor_2D_VisualizationData/Sensor_3_Left ==
  Sensor : Inport
  Angle_Hor_Rel[deg] : Gain
  Angle_ScopeZone_Horizontal[deg] : Gain
  Angle_z_Orientation_Sensor_CoorSys_V[deg] : Gain
  Bus Selector : BusSelector  OutputSignals=Parameters.Sensor_Enable[0Off|1On],Parameters.Sensor_Detection_Mode[1Ray|2Sector],Parameters.Length_ScopeZone[m],Parameters.Pos_Sensor_Apex_CoorSys_V[x;y;z][m],Parameters.Angle_z_Orientation_Sensor_CoorSys_V[deg],Parameters.Angle_ScopeZone_Horizontal[deg],Parameters.SensorIdx[],SensorOutput.Object_ID[],SensorOutput.Distance[m],SensorOutput.Angle_Hor_Rel[deg]
  Distance[m] : Gain
  Length_ScopeZone[m] : Gain
  Object_ID[] : Gain
  Pos_Sensor_Apex_CoorSys_V[x;y;z][m] : Gain
  SensorIdx[] : Gain
  Sensor_Detection_Mode[1Ray|2Sector] : Gain
  Sensor_Enable[0Off|1On] : Gain
  Terminator{,1..9} (10 alike) : Terminator
  wires:
  Bus Selector/3 -> Length_ScopeZone[m]/1  "<Length_ScopeZone[m]>"
  Length_ScopeZone[m]/1 -> Terminator9/1
  Bus Selector/10 -> Angle_Hor_Rel[deg]/1  "<Angle_Hor_Rel[deg]>"
  Bus Selector/9 -> Distance[m]/1  "<Distance[m]>"
  Bus Selector/8 -> Object_ID[]/1  "<Object_ID[]>"
  Bus Selector/7 -> SensorIdx[]/1  "<SensorIdx[]>"
  Bus Selector/6 -> Angle_ScopeZone_Horizontal[deg]/1  "<Angle_ScopeZone_Horizontal[deg]>"
  Bus Selector/5 -> Angle_z_Orientation_Sensor_CoorSys_V[deg]/1  "<Angle_z_Orientation_Sensor_CoorSys_V[deg]>"
  Bus Selector/4 -> Pos_Sensor_Apex_CoorSys_V[x;y;z][m]/1  "<Pos_Sensor_Apex_CoorSys_V[x;y;z][m]>"
  Angle_Hor_Rel[deg]/1 -> Terminator8/1
  Distance[m]/1 -> Terminator7/1
  Object_ID[]/1 -> Terminator6/1
  SensorIdx[]/1 -> Terminator5/1
  Angle_ScopeZone_Horizontal[deg]/1 -> Terminator4/1
  Angle_z_Orientation_Sensor_CoorSys_V[deg]/1 -> Terminator3/1
  Pos_Sensor_Apex_CoorSys_V[x;y;z][m]/1 -> Terminator2/1
  Bus Selector/2 -> Sensor_Detection_Mode[1Ray|2Sector]/1  "<Sensor_Detection_Mode[1Ray|2Sector]>"
  Sensor_Detection_Mode[1Ray|2Sector]/1 -> Terminator1/1
  Sensor_Enable[0Off|1On]/1 -> Terminator/1
  Bus Selector/1 -> Sensor_Enable[0Off|1On]/1  "<Sensor_Enable[0Off|1On]>"
  Sensor/1 -> Bus Selector/1

== system ASM_Traffic_V2X_Complete_Model_2/MDLUserInterface/Environment/MDL_DISP/Traffic/Object_Sensor_2D/Object_Sensor_2D_VisualizationData/Sensor_4_Rear_Left ==
  Sensor : Inport
  Angle_Hor_Rel[deg] : Gain
  Angle_ScopeZone_Horizontal[deg] : Gain
  Angle_z_Orientation_Sensor_CoorSys_V[deg] : Gain
  Bus Selector : BusSelector  OutputSignals=Parameters.Sensor_Enable[0Off|1On],Parameters.Sensor_Detection_Mode[1Ray|2Sector],Parameters.Length_ScopeZone[m],Parameters.Pos_Sensor_Apex_CoorSys_V[x;y;z][m],Parameters.Angle_z_Orientation_Sensor_CoorSys_V[deg],Parameters.Angle_ScopeZone_Horizontal[deg],Parameters.SensorIdx[],SensorOutput.Object_ID[],SensorOutput.Distance[m],SensorOutput.Angle_Hor_Rel[deg]
  Distance[m] : Gain
  Length_ScopeZone[m] : Gain
  Object_ID[] : Gain
  Pos_Sensor_Apex_CoorSys_V[x;y;z][m] : Gain
  SensorIdx[] : Gain
  Sensor_Detection_Mode[1Ray|2Sector] : Gain
  Sensor_Enable[0Off|1On] : Gain
  Terminator{,1..9} (10 alike) : Terminator
  wires:
  Sensor/1 -> Bus Selector/1
  Bus Selector/1 -> Sensor_Enable[0Off|1On]/1  "<Sensor_Enable[0Off|1On]>"
  Sensor_Enable[0Off|1On]/1 -> Terminator/1
  Sensor_Detection_Mode[1Ray|2Sector]/1 -> Terminator1/1
  Bus Selector/2 -> Sensor_Detection_Mode[1Ray|2Sector]/1  "<Sensor_Detection_Mode[1Ray|2Sector]>"
  Pos_Sensor_Apex_CoorSys_V[x;y;z][m]/1 -> Terminator2/1
  Angle_z_Orientation_Sensor_CoorSys_V[deg]/1 -> Terminator3/1
  Angle_ScopeZone_Horizontal[deg]/1 -> Terminator4/1
  SensorIdx[]/1 -> Terminator5/1
  Object_ID[]/1 -> Terminator6/1
  Distance[m]/1 -> Terminator7/1
  Angle_Hor_Rel[deg]/1 -> Terminator8/1
  Bus Selector/4 -> Pos_Sensor_Apex_CoorSys_V[x;y;z][m]/1  "<Pos_Sensor_Apex_CoorSys_V[x;y;z][m]>"
  Bus Selector/5 -> Angle_z_Orientation_Sensor_CoorSys_V[deg]/1  "<Angle_z_Orientation_Sensor_CoorSys_V[deg]>"
  Bus Selector/6 -> Angle_ScopeZone_Horizontal[deg]/1  "<Angle_ScopeZone_Horizontal[deg]>"
  Bus Selector/7 -> SensorIdx[]/1  "<SensorIdx[]>"
  Bus Selector/8 -> Object_ID[]/1  "<Object_ID[]>"
  Bus Selector/9 -> Distance[m]/1  "<Distance[m]>"
  Bus Selector/10 -> Angle_Hor_Rel[deg]/1  "<Angle_Hor_Rel[deg]>"
  Length_ScopeZone[m]/1 -> Terminator9/1
  Bus Selector/3 -> Length_ScopeZone[m]/1  "<Length_ScopeZone[m]>"
